simulink model "Servo_Simulink"  (Simulink 8.1)
settings: Solver=FixedStepDiscrete  StartTime=0.0  StopTime=50.0  FixedStep=0.1  RelTol=1e-3
libraries: jMPClib x2
settings Model: Creator=jocurrie  LastModifiedBy=Jonathan Currie

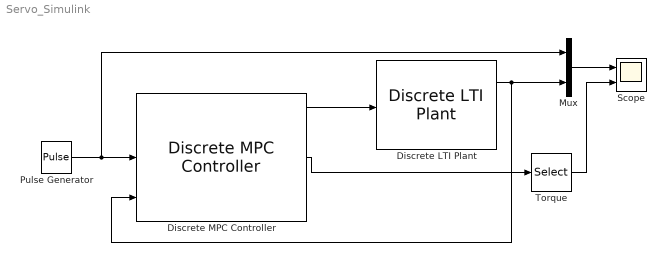
== system Servo_Simulink ==
  Discrete LTI Plant : jMPClib/MPC Blocks/Discrete LTI Plant  jSSobj=Plant
  Discrete MPC Controller : jMPClib/MPC Blocks/Discrete MPC Controller  SIMJMPC=MPC1
  Mux : Mux  Inputs=2
  Pulse Generator : DiscretePulseGenerator  Period=400  PulseWidth=200  SampleTime=0.1
  Scope : Scope  NumInputPorts=2
      settings: YMin=-5~-5  YMax=5~5
  Torque : Selector  InputPortWidth=2  IndexOptions=Index vector (dialog)  Indices=[2]  OutputSizes=1
  wires:
  Discrete MPC Controller/1 -> Discrete LTI Plant/1
  Pulse Generator/1 -> Mux/1, Discrete MPC Controller/2
  Discrete LTI Plant/1 -> Discrete MPC Controller/3, Mux/2
  Mux/1 -> Scope/1
  Discrete MPC Controller/3 -> Torque/1
  Torque/1 -> Scope/2
